simulink model "trab1_questao3_naoLinear"  (R2023b)
settings: Solver=VariableStepAuto  StartTime=0.0  StopTime=30  RelTol=1e-3
libraries: simulink x2
settings Model: Creator=luang  LastModifiedBy=Geovanne
settings SolverCC: AlgebraicLoopSolver=TrustRegion
settings DebuggingCC: UnconnectedInputMsg=warning  UnconnectedOutputMsg=warning  UnconnectedLineMsg=warning
settings ModelReferenceCC: EnableRefExpFcnMdlSchedulingChecks=on

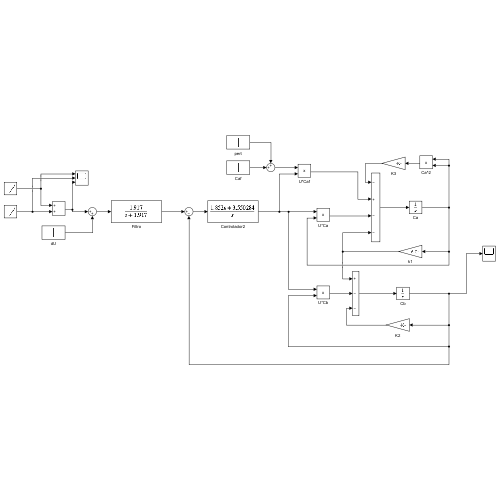
[thumbnail: Simulink's stored preview of the top-level diagram]
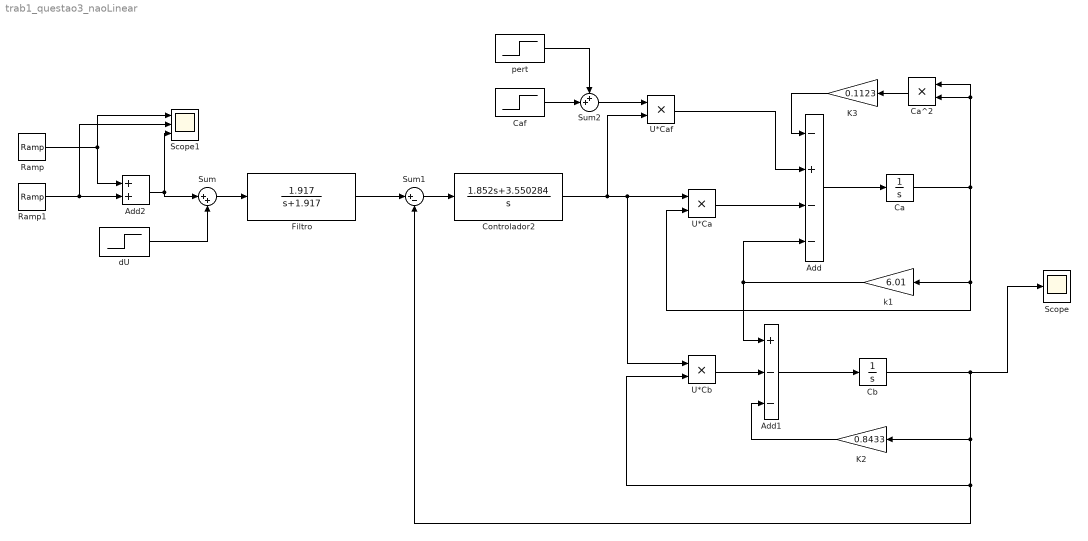
== system trab1_questao3_naoLinear ==
  Add : Sum  Inputs=-+--
  Add1 : Sum  Inputs=+--
  Add2 : Sum
  Ca : Integrator
  Ca^2 : Product
  Caf : Step  Time=0  After=5.1  SampleTime=0
  Cb : Integrator
  Controlador2 : TransferFcn  Numerator=[1.852 3.550284]  Denominator=[1 0]
  Filtro : TransferFcn  Numerator=[1.917]  Denominator=[1 1.917]
  K2 : Gain  Gain=0.8433
  K3 : Gain  Gain=0.1123
  Ramp : simulink/Sources/Ramp  slope=0.5  start=0  InitialOutput=0
  Ramp1 : simulink/Sources/Ramp  slope=-0.5  start=4.69  InitialOutput=0
  Scope : Scope
  Scope1 : Scope  NumInputPorts=3
  Sum : Sum  Inputs=|++
  Sum1 : Sum  Inputs=|+-
  Sum2 : Sum  Inputs=++|
  U*Ca : Product
  U*Caf : Product
  U*Cb : Product
  dU : Step  Time=12  After=0.1  SampleTime=0
  k1 : Gain  Gain=6.01
  pert : Step  Time=20  After=0.3  SampleTime=0
  wires:
  U*Caf/1 -> Add/2
  U*Ca/1 -> Add/3
  Add/1 -> Ca/1
  Ca/1 -> U*Ca/2, k1/1, Ca^2/2, Ca^2/1
  Ca^2/1 -> K3/1
  K3/1 -> Add/1
  K2/1 -> Add1/3
  Cb/1 -> Scope/1, U*Cb/2, Sum1/2, K2/1
  U*Cb/1 -> Add1/2
  Add1/1 -> Cb/1
  k1/1 -> Add1/1, Add/4
  Controlador2/1 -> U*Cb/1, U*Ca/1, U*Caf/2
  Sum/1 -> Filtro/1
  Filtro/1 -> Sum1/1
  Sum1/1 -> Controlador2/1
  dU/1 -> Sum/2
  Caf/1 -> Sum2/2
  pert/1 -> Sum2/1
  Sum2/1 -> U*Caf/1
  Add2/1 -> Sum/1, Scope1/3
  Ramp/1 -> Add2/1, Scope1/1
  Ramp1/1 -> Scope1/2, Add2/2
